simulink model "irradiance"  (R2021a)
settings: Solver=VariableStepAuto  StartTime=0.0  StopTime=10  RelTol=1e-3  AbsTol=1e-3
libraries: simulink x1
settings Model: Creator=Uranus  LastModifiedBy=Uranus
settings SolverCC: AutoScaleAbsTol=off  AlgebraicLoopSolver=TrustRegion
settings DebuggingCC: SymbolicDimsDataTypeCodeGenerationDiagnostic=none  SFMachineParentedDataDiag=warning
settings SFSimCC: CustomCodeUndefinedFunction=UseInterfaceOnly
settings SimscapeCC: SimscapeLogType=all  SimscapeLogSimulationStatistics=on  SimscapeLogDataHistory=10000

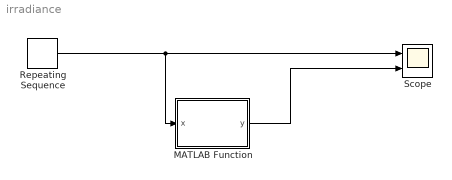
== system irradiance ==
  MATLAB Function : MATLAB Function  TreatAsAtomicUnit=on
  Repeating Sequence : simulink/Sources/Repeating Sequence  rep_seq_t=[0 2 8 10]  rep_seq_y=[0 2 8 10]
  Scope : Scope  NumInputPorts=2
  wires:
  Repeating Sequence/1 -> MATLAB Function/1(x), Scope/1
  MATLAB Function/1(y) -> Scope/2

== matlab function irradiance/MATLAB Function ==
  data: x input; y output
function y = fcn(x)

if x>0 && x<2
    y=x*500;    
elseif x>=2 && x<=8
    y=1000;
elseif x>8 && x<10
    y=5000-500*x;

else 
    y=0;
end
